simulink model "venous_return_curve_model_18017046"  (R2019b)
settings: Solver=VariableStepAuto  StartTime=0.0  StopTime=50  RelTol=1e-3
libraries: simulink x2
settings Model: Creator=User  LastModifiedBy=User

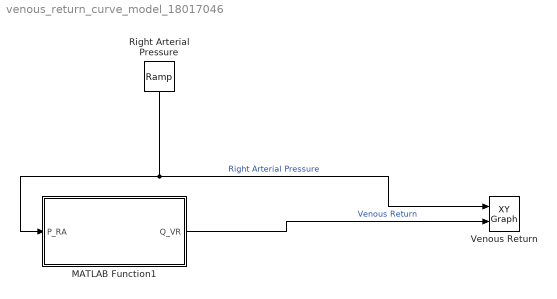
== system venous_return_curve_model_18017046 ==
  MATLAB Function1 : MATLAB Function  TreatAsAtomicUnit=on
  "Right Arterial Pressure " : simulink/Sources/Ramp  slope=1  start=0  InitialOutput=0
  Venous Return : simulink/Sinks/XY Graph  xmin=-20  xmax=50  ymin=-30  ymax=10  st=1
  wires:
  "Right Arterial Pressure "/1 -> Venous Return/1, MATLAB Function1/1(P_RA)  "Right Arterial Pressure"
  MATLAB Function1/1(Q_VR) -> Venous Return/2  "Venous Return"

== matlab function venous_return_curve_model_18017046/MATLAB Function1 ==
  data: P_RA input; Q_VR output
function Q_VR = fcn(P_RA)
P_ms= 7;    % Mean systemic Pressure
R_v= 0.4;   % Ventricular Resistance
R_A= 19.2;  % Atrial Resistance
C_A= 0.028;  % Atrial capacitance
C_V=0.5;    % Ventricular Capacitance
Q_VR = (P_ms-P_RA)/(R_v+(R_A.*C_A+(C_A+C_V)));
